simulink library "INP_SPDWHL_Prep"  (R2024b)
settings: Solver=VariableStepAuto  StartTime=0.0  StopTime=10.0  RelTol=1e-3
undefined symbols (not defined in the file): INP_c_TiSample_s, INP_p_TiTau_s, INP_SPR_p_AccSprOfsFrLe_mps2, INP_SPR_p_AccSprOfsFrRi_mps2, INP_SPR_p_AccSprOfsReLe_mps2, INP_SPR_p_AccSprOfsReRi_mps2, INP_SPR_p_AccSprScaFrLe_na, INP_SPR_p_AccSprScaFrRi_na, INP_SPR_p_AccSprScaReLe_na, INP_SPR_p_AccSprScaReRi_na
libraries: VUT_lib x4
settings Model: Creator=blatak  LastModifiedBy=blatak

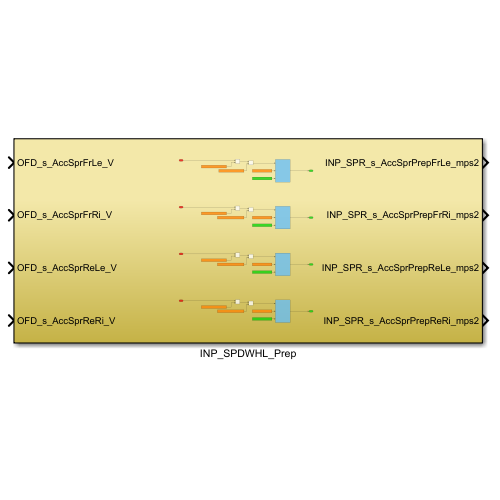
[thumbnail: Simulink's stored preview of the top-level diagram]
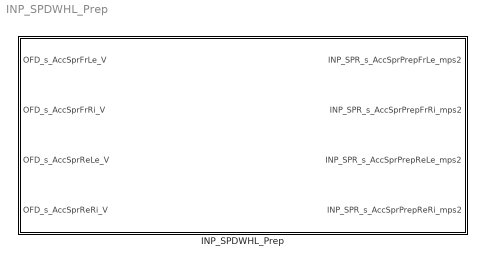
== system INP_SPDWHL_Prep ==
  INP_SPDWHL_Prep : Subsystem

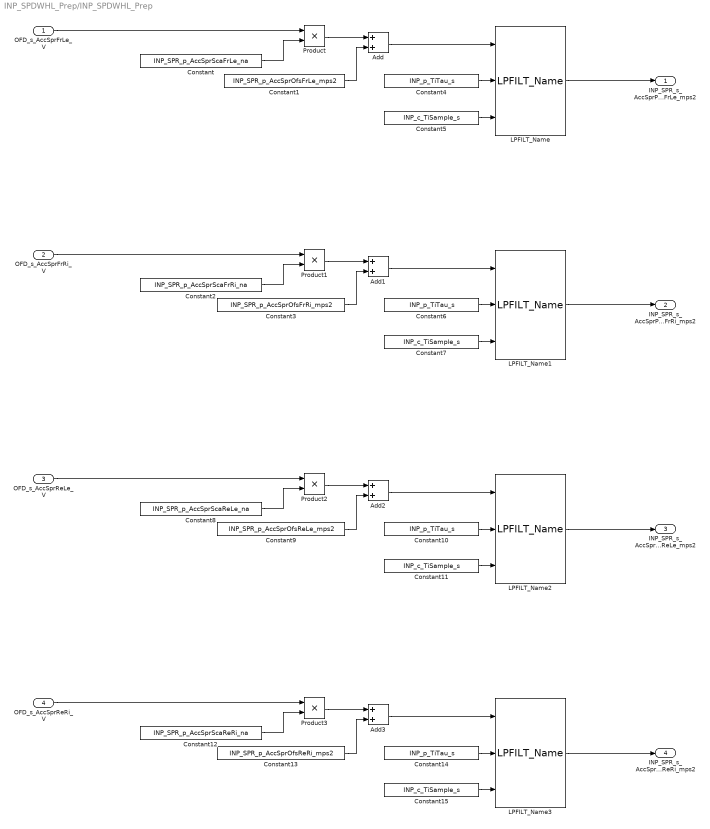
== system INP_SPDWHL_Prep/INP_SPDWHL_Prep ==
  OFD_s_AccSprFrLe_V : Inport
  OFD_s_AccSprFrRi_V : Inport  Port=2
  OFD_s_AccSprReLe_V : Inport  Port=3
  OFD_s_AccSprReRi_V : Inport  Port=4
  Add{,1..3} (4 alike) : Sum
  Constant : Constant  Description=Scaling coefficient to recalculate the electric quantity to the physical one - longitudinal acceleration  Value=INP_SPR_p_AccSprScaFrLe_na
  Constant1 : Constant  Description=Offset to recalculate the electric quantity to the physical one - longitudinal acceleration  Value=INP_SPR_p_AccSprOfsFrLe_mps2
  Constant{4,6,10,14} (4 alike) : Constant  Value=INP_p_TiTau_s
  Constant{5,7,11,15} (4 alike) : Constant  Value=INP_c_TiSample_s
  Constant12 : Constant  Description=Scaling coefficient to recalculate the electric quantity to the physical one - longitudinal acceleration  Value=INP_SPR_p_AccSprScaReRi_na
  Constant13 : Constant  Description=Offset to recalculate the electric quantity to the physical one - longitudinal acceleration  Value=INP_SPR_p_AccSprOfsReRi_mps2
  Constant2 : Constant  Description=Scaling coefficient to recalculate the electric quantity to the physical one - longitudinal acceleration  Value=INP_SPR_p_AccSprScaFrRi_na
  Constant3 : Constant  Description=Offset to recalculate the electric quantity to the physical one - longitudinal acceleration  Value=INP_SPR_p_AccSprOfsFrRi_mps2
  Constant8 : Constant  Description=Scaling coefficient to recalculate the electric quantity to the physical one - longitudinal acceleration  Value=INP_SPR_p_AccSprScaReLe_na
  Constant9 : Constant  Description=Offset to recalculate the electric quantity to the physical one - longitudinal acceleration  Value=INP_SPR_p_AccSprOfsReLe_mps2
  LPFILT_Name{,1..3} (4 alike) : VUT_lib/LPFILT_Name  SystemSampleTime=-1  VariantActivationTime=update diagram  AllowFlexibleInterface=on  Latency=0  AutoFrameSizeCalculation=off
  Product{,1..3} (4 alike) : Product
  INP_SPR_s_AccSprPrepFrLe_mps2 : Outport
  INP_SPR_s_AccSprPrepFrRi_mps2 : Outport  Port=2
  INP_SPR_s_AccSprPrepReLe_mps2 : Outport  Port=3
  INP_SPR_s_AccSprPrepReRi_mps2 : Outport  Port=4
  wires:
  Constant1/1 -> Add/2
  LPFILT_Name1/1 -> INP_SPR_s_AccSprPrepFrRi_mps2/1
  Constant6/1 -> LPFILT_Name1/2
  LPFILT_Name2/1 -> INP_SPR_s_AccSprPrepReLe_mps2/1
  Constant8/1 -> Product2/2
  Constant2/1 -> Product1/2
  Add1/1 -> LPFILT_Name1/1
  Constant15/1 -> LPFILT_Name3/3
  Constant11/1 -> LPFILT_Name2/3
  Constant4/1 -> LPFILT_Name/2
  Add2/1 -> LPFILT_Name2/1
  Product1/1 -> Add1/1
  Constant10/1 -> LPFILT_Name2/2
  OFD_s_AccSprReLe_V/1 -> Product2/1
  Constant12/1 -> Product3/2
  Constant13/1 -> Add3/2
  Add/1 -> LPFILT_Name/1
  OFD_s_AccSprReRi_V/1 -> Product3/1
  OFD_s_AccSprFrRi_V/1 -> Product1/1
  Constant7/1 -> LPFILT_Name1/3
  Constant3/1 -> Add1/2
  Product3/1 -> Add3/1
  Constant5/1 -> LPFILT_Name/3
  Product2/1 -> Add2/1
  Constant9/1 -> Add2/2
  Product/1 -> Add/1
  Constant14/1 -> LPFILT_Name3/2
  LPFILT_Name3/1 -> INP_SPR_s_AccSprPrepReRi_mps2/1
  Add3/1 -> LPFILT_Name3/1
  OFD_s_AccSprFrLe_V/1 -> Product/1
  LPFILT_Name/1 -> INP_SPR_s_AccSprPrepFrLe_mps2/1
  Constant/1 -> Product/2
